simulink model "Sim_ControladorLQR_Kalman"  (R2024a)
settings: Solver=ode15s  StartTime=0.0  StopTime=30  MaxStep=.0001  RelTol=1e-3
values from neighbouring files (symbols this model uses):
  deg_inicial = 15    [Design_LQR_Kalman.m]    (also in DisenControl.m = 5; DisenControlKalman.m)
  h = 0.001    [Design_LQR_Kalman.m]    (also in DisenControl.m; DisenControlKalman.m = 0.0001)
  Kd = dlqr(mG,mH,Q,R)    [Design_LQR_Kalman.m]    (also in DisenControl.m; DisenControlKalman.m)
  mA = mA_con    [Design_LQR_Kalman.m]    (also in DisenControlKalman.m; Param_Project.m = [       0,   1,        0,                 0; Parametros_Proyecto.m = [       0,   1,        0,                 0)
  mB = mB_con    [Design_LQR_Kalman.m]    (also in DisenControlKalman.m; Param_Project.m = [0; Parametros_Proyecto.m = [0)
  mC = mC_con    [Design_LQR_Kalman.m]    (also in DisenControlKalman.m; Param_Project.m = eye(4); Parametros_Proyecto.m = eye(4))
  mC_medido = [1, 0, 0 ... (first row only)    [Design_LQR_Kalman.m]    (also in DisenControlKalman.m)
  mD = mD_con    [Design_LQR_Kalman.m]    (also in DisenControlKalman.m; Param_Project.m = [0; 0; 0; 0]; Parametros_Proyecto.m = [0; 0; 0; 0])
  mG = PlantaD.A    [Design_LQR_Kalman.m]    (also in DisenControl.m; DisenControlKalman.m)
  mH = PlantaD.B    [Design_LQR_Kalman.m]    (also in DisenControl.m; DisenControlKalman.m)
  R_kalman = diag([1e-5, 1e-3])    [Design_LQR_Kalman.m]    (also in DisenControlKalman.m = diag([1e-3, 1e-2]))
undefined symbols (not defined in the file or in its folder): Ld
libraries: simulink x2
settings Model: Creator=isposzax  LastModifiedBy=alen2

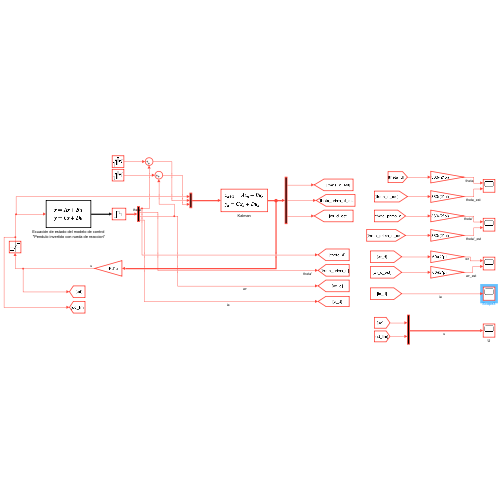
[thumbnail: Simulink's stored preview of the top-level diagram]
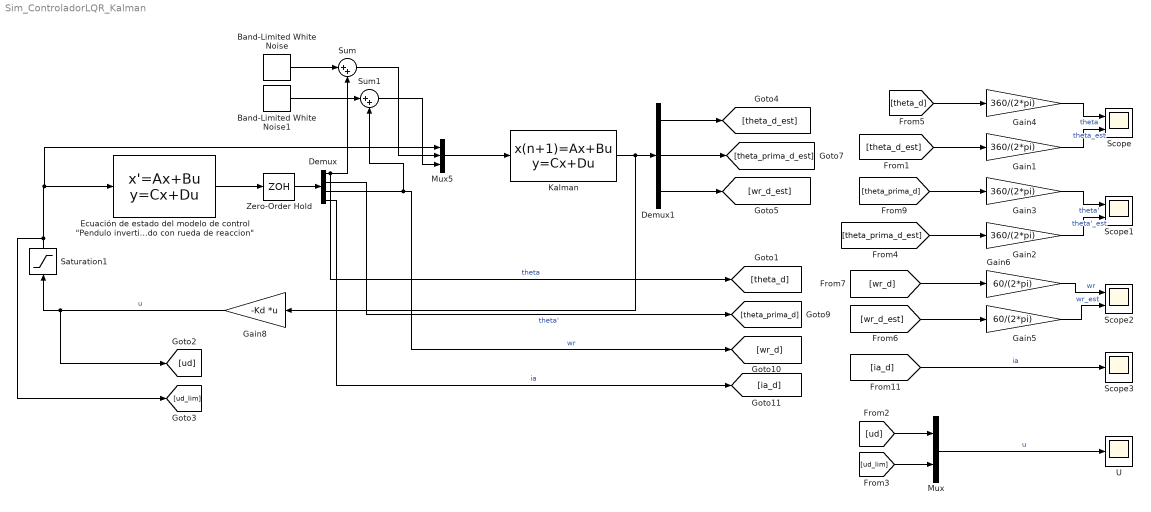
== system Sim_ControladorLQR_Kalman ==
  Band-Limited White Noise : simulink/Sources/Band-Limited White Noise  Cov=R_kalman(1,1) * h  Ts=h  seed=[23341]
  Band-Limited White Noise1 : simulink/Sources/Band-Limited White Noise  Cov=R_kalman(2,2) * h  Ts=h  seed=[87654]
  Demux : Demux
  Demux1 : Demux  Outputs=3
  "Ecuación de estado del modelo de control \"Pendulo invertido con rueda de reaccion\"" : StateSpace  A=mA  B=mB  C=mC  D=mD  InitialCondition=[deg_inicial*pi/180 0 0]
  Gain{1..4} (4 alike) : Gain  Gain=360/(2*pi)
  Gain5 : Gain  Gain=60/(2*pi)
  Gain6 : Gain  Gain=60/(2*pi)
  Gain8 : Gain  Gain=-Kd  Multiplication=Matrix(K*u)
  Kalman : DiscreteStateSpace  A=[mG-Ld*mC_medido]  B=[mH, Ld]  C=eye(size(mG))  D=zeros(3,3)  InitialCondition=[0; 0; 0]  SampleTime=h
  Mux : Mux  Inputs=2
  Mux5 : Mux  Inputs=3
  Saturation1 : Saturate  UpperLimit=12  LowerLimit=-12
  Scope : Scope  NumInputPorts=2
  Scope1 : Scope  NumInputPorts=2
  Scope2 : Scope  NumInputPorts=2
  Scope3 : Scope
  Sum : Sum  Inputs=|++
  Sum1 : Sum  Inputs=|++
  U : Scope
  Zero-Order Hold : ZeroOrderHold  SampleTime=h
  wires:
  Gain4/1 -> Scope/1  "theta"
  Gain3/1 -> Scope1/1  "theta'"
  Gain6/1 -> Scope2/1  "wr"
  Gain8/1 -> [ud], Saturation1/1  "u"
  Demux/1 -> Sum/2, [theta_d]  "theta"
  Demux/2 -> [theta_prima_d]  "theta'"
  Demux/3 -> [wr_d], Sum1/2  "wr"
  Demux/4 -> [ia_d]  "ia"
  Mux/1 -> U/1  "u"
  [theta_d] -> Gain4/1
  Saturation1/1 -> Mux5/1, "Ecuación de estado del modelo de control \"Pendulo invertido con rueda de reaccion\""/1, [ud_lim]
  "Ecuación de estado del modelo de control \"Pendulo invertido con rueda de reaccion\""/1 -> Zero-Order Hold/1
  Mux5/1 -> Kalman/1
  Zero-Order Hold/1 -> Demux/1
  [ud] -> Mux/1
  [ud_lim] -> Mux/2
  [ia_d] -> Scope3/1  "ia"
  [theta_prima_d] -> Gain3/1
  [wr_d] -> Gain6/1
  Kalman/1 -> Gain8/1, Demux1/1
  Demux1/1 -> [theta_d_est]
  Demux1/2 -> [theta_prima_d_est]
  Demux1/3 -> [wr_d_est]
  [theta_d_est] -> Gain1/1
  Gain1/1 -> Scope/2  "theta_est"
  [theta_prima_d_est] -> Gain2/1
  Gain2/1 -> Scope1/2  "theta'_est"
  [wr_d_est] -> Gain5/1
  Gain5/1 -> Scope2/2  "wr_est"
  Band-Limited White Noise/1 -> Sum/1
  Sum/1 -> Mux5/2
  Band-Limited White Noise1/1 -> Sum1/1
  Sum1/1 -> Mux5/3
